simulink model "discrete_10"  (R2021b)
settings: Solver=VariableStepAuto  StartTime=0.0  StopTime=10.0  RelTol=1e-3
undefined symbols (not defined in the file or in its folder): DC, DCM0, DCM1, DCM5, DCS0, DCS1, DCS5, DCT0, DCT1, DCT5, DG, NC, NCM0, NCM1, NCM5, NCS0, NCS1, NCS5, NCT0, NCT1, NCT5, NG
settings Model: Creator=gabri  LastModifiedBy=gabri

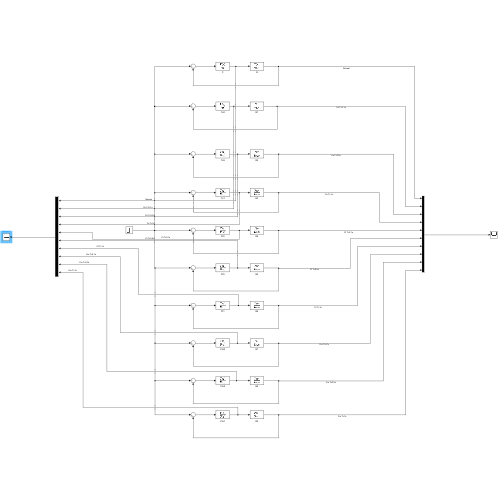
[thumbnail: Simulink's stored preview of the top-level diagram]
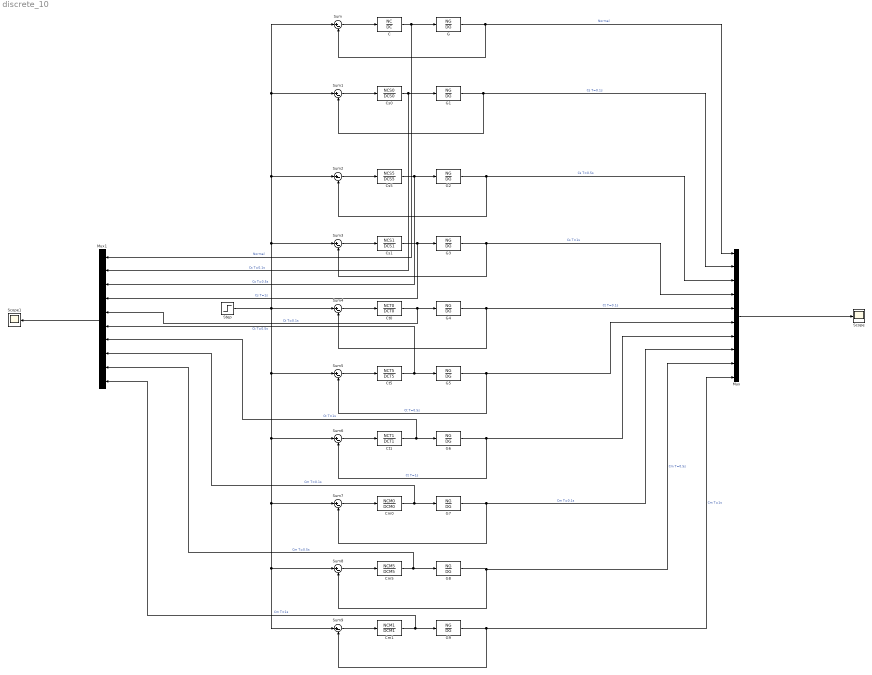
== system discrete_10 ==
  C : TransferFcn  Numerator=NC  Denominator=DC
  Cm0 : DiscreteTransferFcn  Numerator=NCM0  Denominator=DCM0  SampleTime=0.1
  Cm1 : DiscreteTransferFcn  Numerator=NCM1  Denominator=DCM1  SampleTime=1
  Cm5 : DiscreteTransferFcn  Numerator=NCM5  Denominator=DCM5  SampleTime=0.5
  Cs0 : DiscreteTransferFcn  Numerator=NCS0  Denominator=DCS0  SampleTime=0.1
  Cs1 : DiscreteTransferFcn  Numerator=NCS1  Denominator=DCS1  SampleTime=1
  Cs5 : DiscreteTransferFcn  Numerator=NCS5  Denominator=DCS5  SampleTime=0.5
  Ct0 : DiscreteTransferFcn  Numerator=NCT0  Denominator=DCT0  SampleTime=0.1
  Ct1 : DiscreteTransferFcn  Numerator=NCT1  Denominator=DCT1  SampleTime=1
  Ct5 : DiscreteTransferFcn  Numerator=NCT5  Denominator=DCT5  SampleTime=0.5
  G{,1..9} (10 alike) : TransferFcn  Numerator=NG  Denominator=DG
  Mux : Mux  Inputs=10
  Mux1 : Mux  Inputs=10
  Scope : Scope
  Scope1 : Scope
  Step : Step  Time=0  After=10  SampleTime=0
  Sum{,1..9} (10 alike) : Sum  Inputs=|+-
  wires:
  Sum/1 -> C/1
  C/1 -> G/1, Mux1/1  "Normal"
  G/1 -> Mux/1, Sum/2  "Normal"
  Sum1/1 -> Cs0/1
  Cs0/1 -> G1/1, Mux1/2  "Cs T=0.1s"
  G1/1 -> Sum1/2, Mux/2  "Cs T=0.1s"
  Mux/1 -> Scope/1
  Cs5/1 -> Mux1/3, G2/1  "Cs T=0.5s"
  Sum2/1 -> Cs5/1
  G2/1 -> Mux/3, Sum2/2  "Cs T=0.5s"
  Step/1 -> Sum/1, Sum1/1, Sum2/1, Sum3/1, Sum7/1, Sum9/1, Sum8/1, Sum6/1, Sum5/1, Sum4/1
  Cs1/1 -> Mux1/4, G3/1  "Cs T=1s"
  G3/1 -> Sum3/2, Mux/4  "Cs T=1s"
  Sum3/1 -> Cs1/1
  G4/1 -> Sum4/2, Mux/5  "Ct T=0.1s"
  Sum4/1 -> Ct0/1
  Ct0/1 -> Mux1/5, G4/1  "Ct T=0.1s"
  G5/1 -> Mux/6, Sum5/2  "Ct T=0.5s"
  G6/1 -> Mux/7, Sum6/2  "Ct T=1s"
  Sum5/1 -> Ct5/1
  Sum6/1 -> Ct1/1
  Ct5/1 -> Mux1/6, G5/1  "Ct T=0.5s"
  Ct1/1 -> G6/1, Mux1/7  "Ct T=1s"
  G7/1 -> Mux/8, Sum7/2  "Cm T=0.1s"
  G8/1 -> Mux/9, Sum8/2  "Cm T=0.5s"
  Sum7/1 -> Cm0/1
  Sum8/1 -> Cm5/1
  Cm0/1 -> G7/1, Mux1/8  "Cm T=0.1s"
  Cm5/1 -> G8/1, Mux1/9  "Cm T=0.5s"
  Cm1/1 -> Mux1/10, G9/1  "Cm T=1s"
  Sum9/1 -> Cm1/1
  G9/1 -> Sum9/2, Mux/10  "Cm T=1s"
  Mux1/1 -> Scope1/1
